simulink model "TST_Rail_TempLim"  (R2016b)
settings: Solver=FixedStepDiscrete  StartTime=0.0  StopTime=simTime  FixedStep=sampleTime  RelTol=1e-3
values from neighbouring files (symbols this model uses):
  testCase = 1    [initTST_Rail_TempLim_001.m]
libraries: simulink x3, UnitTest_Lib x1
settings Model: Creator=zhengjinyan  LastModifiedBy=zhengjinyan
settings DebuggingCC: SignalRangeChecking=error

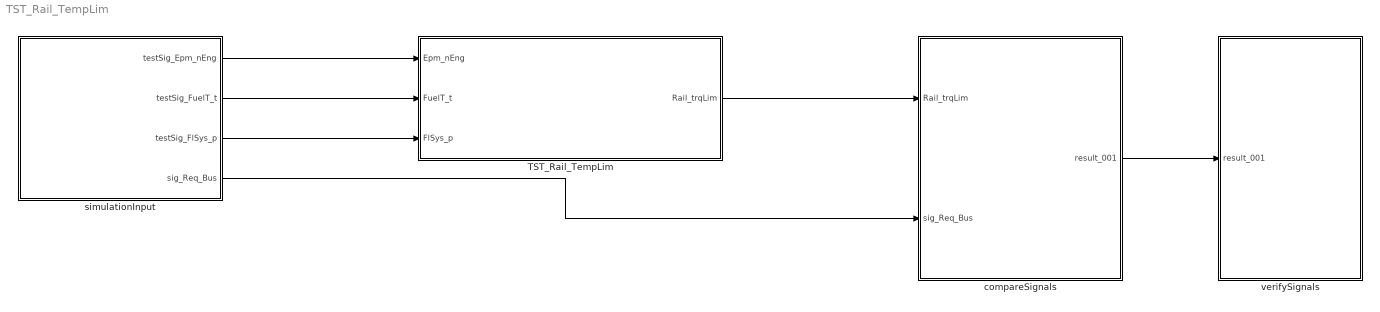
== system TST_Rail_TempLim ==
  TST_Rail_TempLim : Subsystem
  compareSignals : Subsystem
  simulationInput : Subsystem
  verifySignals : Subsystem
  wires:
  simulationInput/1(testSig_Epm_nEng) -> TST_Rail_TempLim/1(Epm_nEng)
  simulationInput/2(testSig_FuelT_t) -> TST_Rail_TempLim/2(FuelT_t)
  simulationInput/3(testSig_FlSys_p) -> TST_Rail_TempLim/3(FlSys_p)
  TST_Rail_TempLim/1(Rail_trqLim) -> compareSignals/1(Rail_trqLim)
  simulationInput/4(sig_Req_Bus) -> compareSignals/2(sig_Req_Bus)
  compareSignals/1(result_001) -> verifySignals/1(result_001)

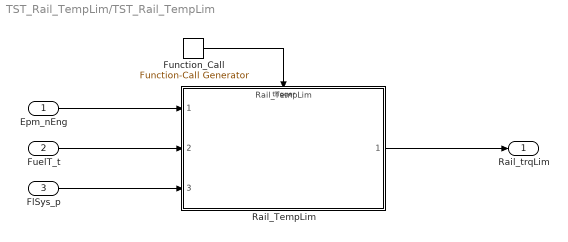
== system TST_Rail_TempLim/TST_Rail_TempLim ==
  Epm_nEng : Inport
  FuelT_t : Inport  Port=2
  FlSys_p : Inport  Port=3
  Function_Call : simulink/Ports & Subsystems/Function-Call Generator  sample_time=sampleTime  numberOfIterations=1
  Rail_TempLim : ModelReference  ModelNameDialog=Rail_TempLim  SimulationMode=Normal  ModelReferenceVersion=1.7  TriggerPortName=function  TriggerPortTriggerType=function-call  TriggerPortStatesWhenEnabling=held
  Rail_trqLim : Outport
  wires:
  Function_Call/1 -> Rail_TempLim/Trigger
  Epm_nEng/1 -> Rail_TempLim/1
  FuelT_t/1 -> Rail_TempLim/2
  FlSys_p/1 -> Rail_TempLim/3
  Rail_TempLim/1 -> Rail_trqLim/1

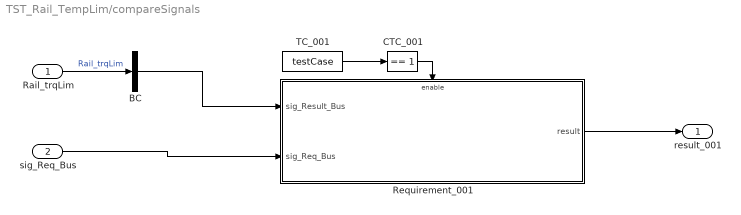
== system TST_Rail_TempLim/compareSignals ==
  Rail_trqLim : Inport
  sig_Req_Bus : Inport  Port=2
  BC : BusCreator  Inputs=1
  CTC_001 : simulink/Logic and Bit Operations/Compare To Constant  relop===  const=1  OutDataTypeStr=boolean
  Requirement_001 : Subsystem
  TC_001 : Constant  Value=testCase
  result_001 : Outport
  wires:
  Rail_trqLim/1 -> BC/1  "Rail_trqLim"
  TC_001/1 -> CTC_001/1
  CTC_001/1 -> Requirement_001/Enable
  sig_Req_Bus/1 -> Requirement_001/2(sig_Req_Bus)
  BC/1 -> Requirement_001/1(sig_Result_Bus)
  Requirement_001/1(result) -> result_001/1

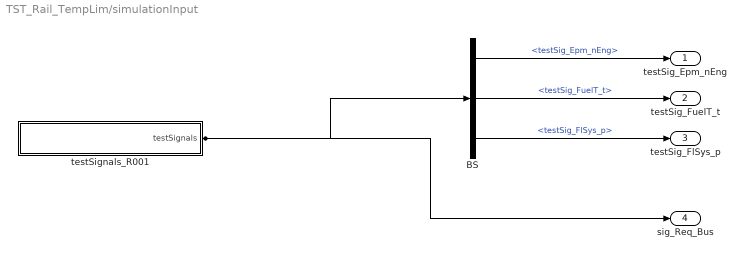
== system TST_Rail_TempLim/simulationInput ==
  BS : BusSelector  OutputSignals=testSig_Epm_nEng,testSig_FuelT_t,testSig_FlSys_p
  testSignals_R001 : Subsystem
  testSig_Epm_nEng : Outport
  testSig_FuelT_t : Outport  Port=2
  testSig_FlSys_p : Outport  Port=3
  sig_Req_Bus : Outport  Port=4
  wires:
  BS/1 -> testSig_Epm_nEng/1  "<testSig_Epm_nEng>"
  BS/2 -> testSig_FuelT_t/1  "<testSig_FuelT_t>"
  BS/3 -> testSig_FlSys_p/1  "<testSig_FlSys_p>"
  testSignals_R001/1(testSignals) -> BS/1, sig_Req_Bus/1

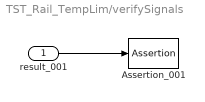
== system TST_Rail_TempLim/verifySignals ==
  result_001 : Inport
  Assertion_001 : Assertion  Enabled=off
  wires:
  result_001/1 -> Assertion_001/1

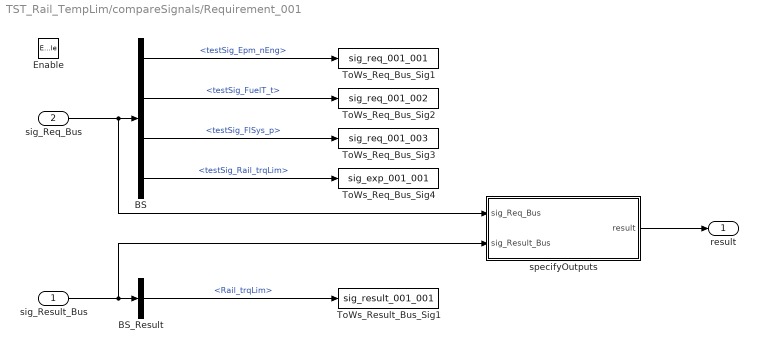
== system TST_Rail_TempLim/compareSignals/Requirement_001 ==
  sig_Result_Bus : Inport
  sig_Req_Bus : Inport  Port=2
  Enable : EnablePort
  BS : BusSelector  OutputSignals=testSig_Epm_nEng,testSig_FuelT_t,testSig_FlSys_p,testSig_Rail_trqLim
  BS_Result : BusSelector  OutputSignals=Rail_trqLim
  ToWs_Req_Bus_Sig1 : ToWorkspace  VariableName=sig_req_001_001  SaveFormat=Structure With Time
  ToWs_Req_Bus_Sig2 : ToWorkspace  VariableName=sig_req_001_002  SaveFormat=Structure With Time
  ToWs_Req_Bus_Sig3 : ToWorkspace  VariableName=sig_req_001_003  SaveFormat=Structure With Time
  ToWs_Req_Bus_Sig4 : ToWorkspace  VariableName=sig_exp_001_001  SaveFormat=Structure With Time
  ToWs_Result_Bus_Sig1 : ToWorkspace  VariableName=sig_result_001_001  SaveFormat=Structure With Time
  specifyOutputs : Subsystem
  result : Outport
  wires:
  sig_Req_Bus/1 -> BS/1, specifyOutputs/1(sig_Req_Bus)
  BS/1 -> ToWs_Req_Bus_Sig1/1  "<testSig_Epm_nEng>"
  BS/2 -> ToWs_Req_Bus_Sig2/1  "<testSig_FuelT_t>"
  BS/3 -> ToWs_Req_Bus_Sig3/1  "<testSig_FlSys_p>"
  BS/4 -> ToWs_Req_Bus_Sig4/1  "<testSig_Rail_trqLim>"
  sig_Result_Bus/1 -> BS_Result/1, specifyOutputs/2(sig_Result_Bus)
  BS_Result/1 -> ToWs_Result_Bus_Sig1/1  "<Rail_trqLim>"
  specifyOutputs/1(result) -> result/1

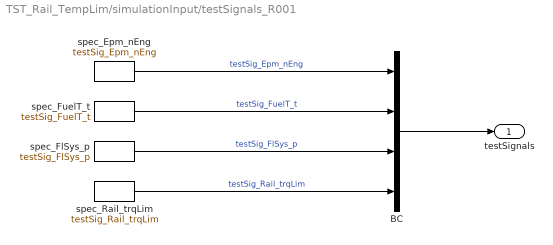
== system TST_Rail_TempLim/simulationInput/testSignals_R001 ==
  BC : BusCreator  Inputs=4
  spec_Epm_nEng : FromWorkspace  VariableName=testSig_Epm_nEng  Interpolate=off  OutputAfterFinalValue=Holding final value
  spec_FlSys_p : FromWorkspace  VariableName=testSig_FlSys_p  Interpolate=off  OutputAfterFinalValue=Holding final value
  spec_FuelT_t : FromWorkspace  VariableName=testSig_FuelT_t  Interpolate=off  OutputAfterFinalValue=Holding final value
  spec_Rail_trqLim : FromWorkspace  VariableName=testSig_Rail_trqLim  Interpolate=off  OutputAfterFinalValue=Holding final value
  testSignals : Outport
  wires:
  BC/1 -> testSignals/1
  spec_Epm_nEng/1 -> BC/1  "testSig_Epm_nEng"
  spec_FuelT_t/1 -> BC/2  "testSig_FuelT_t"
  spec_FlSys_p/1 -> BC/3  "testSig_FlSys_p"
  spec_Rail_trqLim/1 -> BC/4  "testSig_Rail_trqLim"

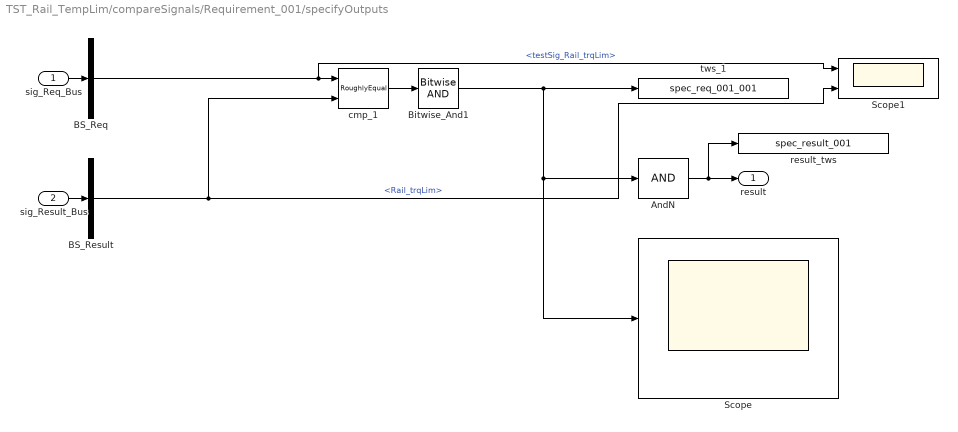
== system TST_Rail_TempLim/compareSignals/Requirement_001/specifyOutputs ==
  sig_Req_Bus : Inport
  sig_Result_Bus : Inport  Port=2
  AndN : Logic  Inputs=1
  BS_Req : BusSelector  OutputSignals=testSig_Rail_trqLim
  BS_Result : BusSelector  OutputSignals=Rail_trqLim
  Bitwise_And1 : simulink/Logic and Bit Operations/Bitwise Operator  logicop=AND  UseBitMask=off  BitMask=bin2dec('11011001')  BitMaskRealWorld=Stored Integer
  Scope : Scope
  Scope1 : Scope  NumInputPorts=2
  cmp_1 : UnitTest_Lib/RoughlyEqual  slope=0.2
  result_tws : ToWorkspace  VariableName=spec_result_001
  tws_1 : ToWorkspace  VariableName=spec_req_001_001
  result : Outport
  wires:
  sig_Req_Bus/1 -> BS_Req/1
  sig_Result_Bus/1 -> BS_Result/1
  AndN/1 -> result/1, result_tws/1
  BS_Req/1 -> cmp_1/1, Scope1/1  "<testSig_Rail_trqLim>"
  BS_Result/1 -> cmp_1/2, Scope1/2  "<Rail_trqLim>"
  cmp_1/1 -> Bitwise_And1/1
  Bitwise_And1/1 -> AndN/1, Scope/1, tws_1/1
